simulink model "reference_tracking"  (R2022a)
settings: Solver=VariableStepAuto  StartTime=0.0  StopTime=500  RelTol=1e-3
values from neighbouring files (symbols this model uses):
  sys2 = ss(Ar,Br,Cr,Dr, "statename", states, "inputname", inputs, "outputname", outputs)    [shaped_model.m]
undefined symbols (not defined in the file or in its folder): K2
settings Model: Creator=ritvi  LastModifiedBy=ritvi

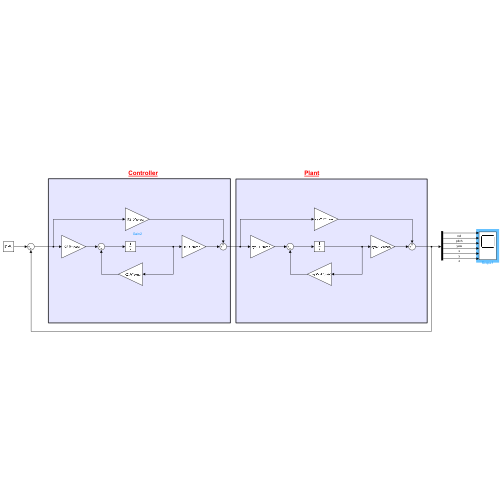
[thumbnail: Simulink's stored preview of the top-level diagram]
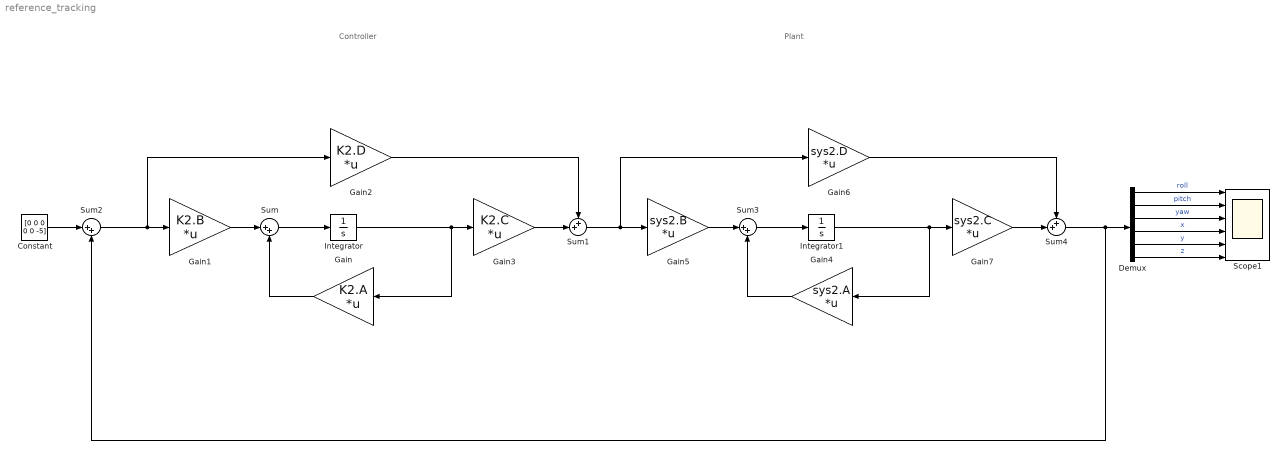
== system reference_tracking ==
  note: Controller
  note: Plant
  Constant : Constant  Value=[0 0 0 0 0 -5]  VectorParams1D=off
  Demux : Demux  Outputs=6
  Gain : Gain  Gain=K2.A  Multiplication=Matrix(K*u) (u vector)
  Gain1 : Gain  Gain=K2.B  Multiplication=Matrix(K*u) (u vector)
  Gain2 : Gain  Gain=K2.D  Multiplication=Matrix(K*u) (u vector)
  Gain3 : Gain  Gain=K2.C  Multiplication=Matrix(K*u) (u vector)
  Gain4 : Gain  Gain=sys2.A  Multiplication=Matrix(K*u) (u vector)
  Gain5 : Gain  Gain=sys2.B  Multiplication=Matrix(K*u) (u vector)
  Gain6 : Gain  Gain=sys2.D  Multiplication=Matrix(K*u) (u vector)
  Gain7 : Gain  Gain=sys2.C  Multiplication=Matrix(K*u) (u vector)
  Integrator : Integrator
  Integrator1 : Integrator
  Scope1 : Scope  NumInputPorts=6
  Sum : Sum  Inputs=|++
  Sum1 : Sum  Inputs=++|
  Sum2 : Sum  Inputs=|++
  Sum3 : Sum  Inputs=|++
  Sum4 : Sum  Inputs=++|
  wires:
  Sum/1 -> Integrator/1
  Integrator/1 -> Gain3/1, Gain/1
  Gain/1 -> Sum/2
  Gain1/1 -> Sum/1
  Gain3/1 -> Sum1/2
  Gain2/1 -> Sum1/1
  Gain4/1 -> Sum3/2
  Sum3/1 -> Integrator1/1
  Gain5/1 -> Sum3/1
  Integrator1/1 -> Gain7/1, Gain4/1
  Gain6/1 -> Sum4/1
  Gain7/1 -> Sum4/2
  Sum1/1 -> Gain6/1, Gain5/1
  Sum4/1 -> Demux/1, Sum2/2
  Constant/1 -> Sum2/1
  Sum2/1 -> Gain2/1, Gain1/1
  Demux/1 -> Scope1/1  "roll"
  Demux/2 -> Scope1/2  "pitch"
  Demux/3 -> Scope1/3  "yaw"
  Demux/4 -> Scope1/4  "x"
  Demux/5 -> Scope1/5  "y"
  Demux/6 -> Scope1/6  "z"
